simulink model "inverternewupdated"  (R2018b)
settings: Solver=VariableStepAuto  StartTime=0.0  StopTime=0.1  RelTol=1e-3
libraries: powerlib x14, simulink x4
settings Model: Creator=Prathyum.G  LastModifiedBy=Prathyum.G

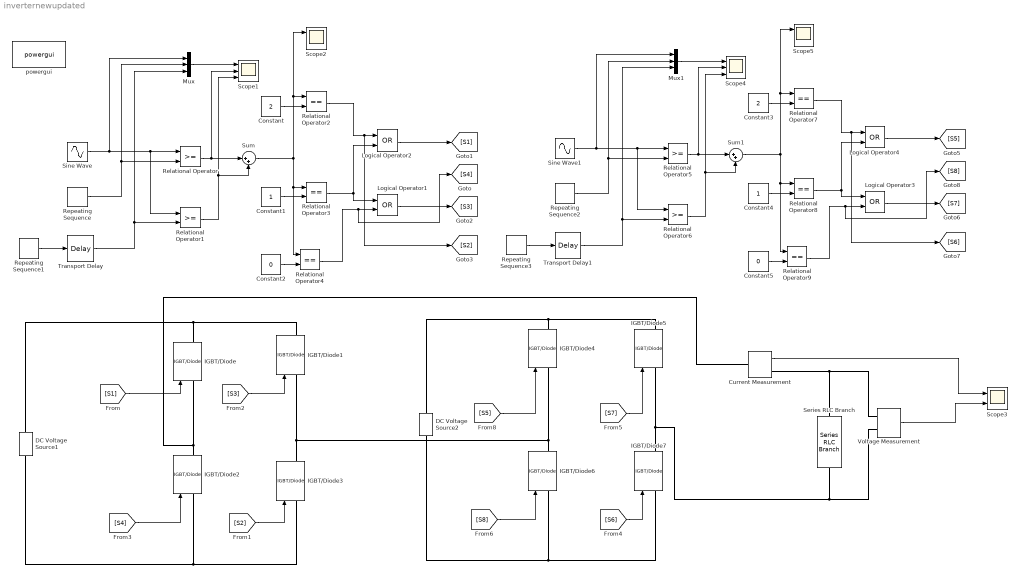
== system inverternewupdated ==
  Constant : Constant  Value=2
  Constant1 : Constant
  Constant2 : Constant  Value=0
  Constant3 : Constant  Value=2
  Constant4 : Constant
  Constant5 : Constant  Value=0
  Current Measurement : powerlib/Measurements/Current Measurement  PhasorSimulation=off  OutputType=Complex  PSBequivalent=0
  DC Voltage Source1 : powerlib/Electrical Sources/DC Voltage Source  Amplitude=100  Measurements=Voltage
  DC Voltage Source2 : powerlib/Electrical Sources/DC Voltage Source  Amplitude=100  Measurements=Voltage
  IGBT/Diode{,1..7} (8 alike) : powerlib/Power Electronics/IGBT//Diode  Ron=1e-3  Rs=1e5  Cs=inf  Measurements=on
  Logical Operator{1..4} (4 alike) : Logic  Operator=OR  AllPortsSameDT=off  OutDataTypeStr=boolean
  Mux : Mux  Inputs=3
  Mux1 : Mux  Inputs=3
  Relational Operator{,1,5..6} (4 alike) : RelationalOperator  OutDataTypeStr=boolean  RndMeth=Simplest
  Relational Operator{2..4,7..9} (6 alike) : RelationalOperator  Operator===  OutDataTypeStr=boolean  RndMeth=Simplest
  Repeating Sequence : simulink/Sources/Repeating Sequence  rep_seq_t=[0 1 2 3 4]*1/40000  rep_seq_y=[0 1 0 -1 0]
  Repeating Sequence1 : simulink/Sources/Repeating Sequence  rep_seq_t=[0 1 2 3 4]*1/40000  rep_seq_y=[0 1 0 -1 0]
  Repeating Sequence2 : simulink/Sources/Repeating Sequence  rep_seq_t=[0 1 2 3 4]*1/40000  rep_seq_y="[1 0 -1  0 1]"
  Repeating Sequence3 : simulink/Sources/Repeating Sequence  rep_seq_t=[0 1 2 3 4]*1/40000  rep_seq_y="[1 0 -1  0 1]"
  Scope{1..2,4..5} (4 alike) : Scope  NumInputPorts=3
  Scope3 : Scope  NumInputPorts=2
  Series RLC Branch : powerlib/Elements/Series RLC Branch  LConnTagsString=__new0  RConnTagsString=__new0  BranchType=RC  Resistance=100  Inductance=1e-3  SetiL0=off  InitialCurrent=0  Capacitance=1e-6  Setx0=off  InitialVoltage=0  Measurements=None
  Sine Wave : Sin  Frequency=2*pi*50  SampleTime=0
  Sine Wave1 : Sin  Frequency=2*pi*50  Phase=pi/2  SampleTime=0
  Sum : Sum  Inputs=|++
  Sum1 : Sum  Inputs=|++
  Transport Delay : TransportDelay  DelayTime=1e-6  InitialOutput=1e-6
  Transport Delay1 : TransportDelay  DelayTime=1.5e-6  InitialOutput=1.5e-6
  Voltage Measurement : powerlib/Measurements/Voltage Measurement  PhasorSimulation=off  OutputType=Complex  PSBequivalent=0
  powergui : powerlib/powergui  Priority=1  SimulationMode=Discrete  SampleTime=1e-06  frequency=60  Iterations=50  frequencyindice=0  Pbase=100e6  ErrMax=1e-4  UnitsV=kV  UnitsW=MW  buscounter=0  FunctionMessages=off  echomessages=off  EnableUseOfTLC=off  CurrentSourceSwitches=off  DisableSnubberDevices=off  DisableRonSwitches=off  DisableVfSwitches=off  DisplayEquations=off  SolverType=Tustin/Backward Euler (TBE)  Interpol=off  ExternalGateDelay=off  methode=off  Ts=100  x0status=blocks  SPID=on  SwTol=0  HookPort=off  RestoreLinks=warning  ResistiveCurrentMeasurement=off  Frange=[0:2:500]  Ylog=off  Xlog=on  ShowGrid=off  save=off  variable=ZData  structure=0  ZoomFFT=off  StartTime=0.0  cycles=1  DisplayStyle=1  fundamental=60  FreqAxis=off  MaxFrequency=1000  frequencyindicesteady=1  RmsSteady=1  display=off
  wires:
  [S1] -> IGBT/Diode/1
  [S3] -> IGBT/Diode1/1
  [S2] -> IGBT/Diode3/1
  [S4] -> IGBT/Diode2/1
  Current Measurement/1 -> Scope3/1
  [S7] -> IGBT/Diode5/1
  [S5] -> IGBT/Diode4/1
  [S6] -> IGBT/Diode7/1
  [S8] -> IGBT/Diode6/1
  Voltage Measurement/1 -> Scope3/2
  Constant/1 -> Relational Operator2/2
  Transport Delay/1 -> Relational Operator1/2, Mux/3
  Constant1/1 -> Relational Operator3/2
  Relational Operator4/1 -> [S4], Logical Operator1/2
  Sum/1 -> Scope2/1, Relational Operator2/1, Relational Operator4/1, Relational Operator3/1
  Repeating Sequence/1 -> Relational Operator/2, Mux/2
  Logical Operator1/1 -> [S3]
  Relational Operator1/1 -> Sum/2, Scope1/3
  Sine Wave/1 -> Mux/1, Relational Operator1/1, Relational Operator/1
  Constant2/1 -> Relational Operator4/2
  Mux/1 -> Scope1/1
  Relational Operator2/1 -> [S2], Logical Operator2/1
  Relational Operator/1 -> Sum/1, Scope1/2
  Repeating Sequence1/1 -> Transport Delay/1
  Relational Operator3/1 -> Logical Operator2/2, Logical Operator1/1
  Logical Operator2/1 -> [S1]
  Constant4/1 -> Relational Operator8/2
  Logical Operator3/1 -> [S7]
  Constant5/1 -> Relational Operator9/2
  Sum1/1 -> Scope5/1, Relational Operator7/1, Relational Operator9/1, Relational Operator8/1
  Relational Operator5/1 -> Sum1/1, Scope4/2
  Relational Operator9/1 -> [S8], Logical Operator3/2
  Relational Operator6/1 -> Sum1/2, Scope4/3
  Logical Operator4/1 -> [S5]
  Relational Operator7/1 -> [S6], Logical Operator4/1
  Repeating Sequence2/1 -> Relational Operator5/2, Mux1/2
  Relational Operator8/1 -> Logical Operator4/2, Logical Operator3/1
  Constant3/1 -> Relational Operator7/2
  Mux1/1 -> Scope4/1
  Transport Delay1/1 -> Relational Operator6/2, Mux1/3
  Sine Wave1/1 -> Mux1/1, Relational Operator6/1, Relational Operator5/1
  Repeating Sequence3/1 -> Transport Delay1/1
  connections:
  IGBT/Diode2/RConn1 -- IGBT/Diode/LConn1 -- Current Measurement/LConn1
  IGBT/Diode/RConn1 -- IGBT/Diode1/RConn1 -- DC Voltage Source1/LConn1
  DC Voltage Source1/RConn1 -- IGBT/Diode2/LConn1 -- IGBT/Diode3/LConn1
  IGBT/Diode7/LConn1 -- IGBT/Diode6/LConn1 -- DC Voltage Source2/RConn1
  IGBT/Diode5/RConn1 -- IGBT/Diode4/RConn1 -- DC Voltage Source2/LConn1
  IGBT/Diode7/RConn1 -- Series RLC Branch/RConn1 -- Voltage Measurement/LConn2 -- IGBT/Diode5/LConn1
  IGBT/Diode3/RConn1 -- IGBT/Diode1/LConn1 -- IGBT/Diode4/LConn1 -- IGBT/Diode6/RConn1
  Series RLC Branch/LConn1 -- Voltage Measurement/LConn1 -- Current Measurement/RConn1
